simulink model "PlanControlZW_cs"  (R2020a)
settings: Solver=VariableStepAuto  StartTime=0.0  StopTime=100  FixedStep=1/1000  RelTol=1e-3
PreLoadFcn:
  | mbxruntime.callbacks.PreLoadFcn(bdroot);
PostLoadFcn:
  | mbxruntime.callbacks.PostLoadFcn(bdroot);
InitFcn:
  | mbxruntime.callbacks.InitFcn(bdroot);
StartFcn:
  | mbxruntime.callbacks.StartFcn(bdroot);
StopFcn:
  | mbxruntime.callbacks.StopFcn(bdroot);
model workspace (MAT data in the model file):
  mbox_table : object (value not decoded)
  model_closed = 0
  sim_status = 0
values from neighbouring files (symbols this model uses):
  c_factor = 43.75    [emplanner_init.m]
  cf = -175016    [emplanner_init.m]
  cr = -130634    [emplanner_init.m]
  global_path_x = [-2.22044604925e-16 0.999382255067 1.99750536558 2.99435224935 3.98991712279 4.98419835808 5.97719585569 6.96891007764 7.95934169183 8.94849144113 9.93636009523 10.9229484329 ... (501 elements, 501x1)]    [global_Path.mat]
  global_path_y = [-1.75 -1.75 -1.75 -1.75 -1.75 -1.75 -1.75 -1.75 -1.75 -1.75 -1.75 -1.75 ... (501 elements, 501x1)]    [global_Path.mat]
  KD_PID_distance = 0.0    (= 0)    [emplanner_init.m]
  KD_PID_speed = 0    [emplanner_init.m]
  KI_PID_distance = 0.0    (= 0)    [emplanner_init.m]
  KI_PID_speed = 0    [emplanner_init.m]
  KP_PID_distance = 0.5    [emplanner_init.m]
  KP_PID_speed = 1.8    [emplanner_init.m]
  la = 1.265    [emplanner_init.m]
  lb = 2.947-1.265    (= 1.682)    [emplanner_init.m]
  LQR_K1 = k(:,1)'    [emplanner_init.m]
  LQR_K2 = k(:,2)'    [emplanner_init.m]
  LQR_K3 = k(:,3)'    [emplanner_init.m]
  LQR_K4 = k(:,4)'    [emplanner_init.m]
  m = 2020    [emplanner_init.m]
  rack_displacement = [-39.14 , -37.2 , -35.29 , -33.43 , -31.6 , -29.81 , -28.06 , -26.34 , -24.66 ,      -23.01 , -21.38 , -19.79 , -18.23 , -16.69 , -15.18 , -13.7 , -12.23 , -10.8 , -9.38 , -7.98 ,     -6.61 , -5.25 , -3.91 , -2.59 , -1.29 , 0 , 1.27 , 2.54 , 3.78 , 5.02 , 6.24 , 7.46 , 8.66 ,      9.86 , 11.05 , 12.24 , 13.41 , 14.59 , 15.76 , 16.92 , 18.09 , 19.25 , 20.42 , 21.59 , 22.76 ,      23.93 , 25.11 , 26 ...(+26 chars)    [emplanner_init.m]
  refrence_path_x = [2.22044604925e-16 0.999382255067 1.99750536558 2.99435224935 3.98991712279 4.98419835808 5.97719585569 6.96891007764 7.95934169183 8.94849144113 9.93636009523 10.9229484329 ... (501 elements, 501x1)]    [refrence_path_two.mat]
  refrence_path_y = [1.75 1.75 1.75 1.75 1.75 1.75 1.75 1.75 1.75 1.75 1.75 1.75 ... (501 elements, 501x1)]    [refrence_path_two.mat]
  right_wheel_ground = [-70 ,-67.2 , -64.4 , -61.6 , -58.8 , -56 , -53.2 , -50.4 , -47.6 , -44.8 , -42 ,      -39.2 , -36.4 , -33.6 , -30.8 , -28 , -25.2 , -22.4 , -19.6 , -16.8 , -14 , -11.2 , -8.4 , -5.6 ,      -2.8 , 0 , 2.8 , 5.6 , 8.4 , 11.2 , 14 , 16.8 , 19.6 , 22.4 , 25.2 , 28 , 30.8 , 33.6 , 36.4 ,      39.2 , 42 , 44.8 , 47.6 , 50.4 , 53.2 , 56 , 58.8 , 61.6 , 64.4 , 67.2 , 70 ]    [emplanner_init.m]
  vx_break_point = zeros(1,5000)    [emplanner_init.m]
undefined symbols (not defined in the file or in its folder): aubr, DiscIntNeverNeededParam, tablebr, vubr
libraries: PreScanSimulinkLibrary x34, simulink_extras x5, Solver_SF x1
(part 10 of 10)

== matlab function PlanControlZW_cs/Audi_A8_Sedan_1/decision&planning module/EM Planner/speed decision with dynamic planning(dp) ==
  data: obs_st_s_in_set input; dp_speed_s output; obs_st_s_out_set input; obs_st_t_in_set input; obs_st_t_out_set input; dp_speed_t output; reference_speed_unlimit input; w_cost_ref_speed input; w_cost_accel input; w_cost_obs input; plan_start_s_dot input
function [dp_speed_s,dp_speed_t] = fcn(obs_st_s_in_set,obs_st_s_out_set,obs_st_t_in_set,obs_st_t_out_set,reference_speed_unlimit...
    ,w_cost_ref_speed,w_cost_accel,w_cost_obs,plan_start_s_dot)
% 速度动态规划
% 时间从0到8开始规划，最多8秒
% s的范围从0开始到路径规划的path的总长度为止
% 为了减少算力 采用非均匀采样，s越小的越密，越大的越稀疏

s_list = [0:0.5:4.5,...
          5.5:1:14.5,...
          16:1.5:29.5,...
          32:2.5:54.5];
% t 采用均匀采样每 0.5s采样一个点
t_list = 0.5:0.5:8;
% 声明st代价矩阵，表示从起点开始到(i,j)点的最小代价为dp_st_cost(i,j)
% s 采样40个 t 采样 16个 一共是 40 * 16
dp_st_cost = ones(40,16) * inf; % 首先初始化为无穷大
% dp_st_s_dot，表示从起点开始到(i,j)点的最优路径的末速度
dp_st_s_dot = zeros(40,16);
% 需要一个矩阵保持最优路径的前一个节点方便回溯
% dp_st_node(i,j) 表示位置为(i,j)的节点中，最优的上一层节点的行号为dp_st_node(i,j)
dp_st_node = zeros(40,16);
% 计算从dp起点到第一列的cost
for i = 1:length(s_list)
    dp_st_cost(i,1) = CalcDpCost(0,0,i,1,obs_st_s_in_set,obs_st_s_out_set,obs_st_t_in_set,obs_st_t_out_set,...
    w_cost_ref_speed,reference_speed_unlimit,w_cost_accel,w_cost_obs,plan_start_s_dot,s_list,t_list,dp_st_s_dot);
    % 计算第一列所有节点的的s_dot，并存储到dp_st_s_dot中
    % 第一列的前一个节点只有起点，起点的s t 都是0
    [s_end,t_end] = CalcSTCoordinate(i,1,s_list,t_list);
    dp_st_s_dot(i,1) = s_end / t_end;
end
% 动态规划主程序
for i = 2:length(t_list)
    % i 为列循环
    for j = 1:length(s_list)
        % j 为行循环
        % 当前行为 j 列为 i
        cur_row = j;
        cur_col = i;
        % 遍历前一列
        for k = 1:length(s_list)
            pre_row = k;
            pre_col = i - 1;
            % 计算边的代价 其中起点为pre_row,pre_col 终点为cur_row cur_col
            cost_temp = CalcDpCost(pre_row,pre_col,cur_row,cur_col,obs_st_s_in_set,obs_st_s_out_set,...
                obs_st_t_in_set,obs_st_t_out_set,w_cost_ref_speed,reference_speed_unlimit,w_cost_accel,w_cost_obs,...
                plan_start_s_dot,s_list,t_list,dp_st_s_dot);
            if cost_temp + dp_st_cost(pre_row,pre_col) < dp_st_cost(cur_row,cur_col)
                dp_st_cost(cur_row,cur_col) = cost_temp + dp_st_cost(pre_row,pre_col);
                % 计算最优的s_dot
                [s_start,t_start] = CalcSTCoordinate(pre_row,pre_col,s_list,t_list);
                [s_end,t_end] = CalcSTCoordinate(cur_row,cur_col,s_list,t_list);
                dp_st_s_dot(cur_row,cur_col) = (s_end - s_start) / (t_end - t_start);
                % 将最短路径的前一个节点的行号记录下来
                dp_st_node(cur_row,cur_col) = pre_row;
            end      
        end
    end
end
% 输出初始化
dp_speed_s = ones(length(t_list),1) * nan;
dp_speed_t = dp_speed_s;
% 找到dp_node_cost 上边界和右边界代价最小的节点
min_cost = inf;
min_row = inf;
min_col = inf;
% for i = 1:length(s_list)
%     % 遍历右边界
%     if dp_st_cost(i,length(t_list)) <= min_cost
%         min_cost = dp_st_cost(i,length(t_list));
%         min_row = i;
%         min_col = length(t_list);
%     end
% end

for j = 1:length(t_list)-5
    % 遍历上边界
    if dp_st_cost(1,j) <= min_cost
        min_cost = dp_st_cost(1,j);
        min_row = 1;
        min_col = j;
    end
end
% 这里要注意，虽然我们在t上每0.5s采样一个时间，采了16个点，但是min_col 未必等于16
% 也就是说动态规划的最优解的时间未必是8秒
% 所以我们动态规划最后的输出s t 不一定是写满
% 先把终点的ST输出出来
[dp_speed_s(min_col),dp_speed_t(min_col)] = CalcSTCoordinate(min_row,min_col,s_list,t_list);
% 反向回溯
while min_col ~= 1
    pre_row = dp_st_node(min_row,min_col);
    pre_col = min_col - 1;
    [dp_speed_s(pre_col),dp_speed_t(pre_col)] = CalcSTCoordinate(pre_row,pre_col,s_list,t_list);
    min_row = pre_row;
    min_col = pre_col;
end


end

function cost = CalcDpCost(row_start,col_start,row_end,col_end,obs_st_s_in_set,obs_st_s_out_set,obs_st_t_in_set,obs_st_t_out_set,...
    w_cost_ref_speed,reference_speed,w_cost_accel,w_cost_obs,plan_start_s_dot,s_list,t_list,dp_st_s_dot)
    % 该函数将计算链接两个节点之间边的代价
    % 输入：边的起点的行列号row_start,col_start 边的终点行列号row_end,col_end
          % 障碍物st信息obs_st_s_in_set,obs_st_s_out_set,obs_st_t_in_set,obs_st_t_out_set
          % 推荐速度代价权重w_cost_ref_speed,加速度代价权重w_cost_accel,障碍物代价权重w_cost_obs
          % 推荐速度reference_speed
          % 拼接起点的速度plan_start_s_dot
          % s_list,t_list 采样距离
          % dp_st_s_dot 用于计算加速度
    % 首先计算终点的st坐标
    [s_end,t_end] = CalcSTCoordinate(row_end,col_end,s_list,t_list);
    % 规定起点的行列号为0 
    if row_start == 0
        % 边的起点为dp的起点
        s_start = 0;
        t_start = 0;
        s_dot_start = plan_start_s_dot;
    else
        % 边的起点不是dp的起点
        [s_start,t_start] = CalcSTCoordinate(row_start,col_start,s_list,t_list);
        s_dot_start = dp_st_s_dot(row_start,col_start);
    end
    cur_s_dot = (s_end - s_start) / (t_end - t_start);
    cur_s_dot2 = (cur_s_dot - s_dot_start)/(t_end - t_start);
    % 计算推荐速度代价
    cost_ref_speed = w_cost_ref_speed * (cur_s_dot - reference_speed)^2;
    % 计算加速度代价，这里注意，加速度不能超过车辆动力学上下限
    if cur_s_dot2 < 4 && cur_s_dot2 > -6
        cost_accel = w_cost_accel * cur_s_dot2^2;
    else
        % 超过车辆动力学限制，代价会增大很多倍
        cost_accel = 100000 * w_cost_accel * cur_s_dot2^2;
    end
    cost_obs = CalcObsCost(s_start,t_start,s_end,t_end,obs_st_s_in_set,obs_st_s_out_set,obs_st_t_in_set,obs_st_t_out_set,w_cost_obs);
    cost = cost_obs + cost_accel + cost_ref_speed;
end

function obs_cost = CalcObsCost(s_start,t_start,s_end,t_end,obs_st_s_in_set,obs_st_s_out_set,obs_st_t_in_set,obs_st_t_out_set,w_cost_obs)
% 该函数将计算边的障碍物代价
% 输入：边的起点终点s_start,t_start,s_end,t_end
%       障碍物信息 obs_st_s_in_set,obs_st_s_out_set,obs_st_t_in_set,obs_st_t_out_set
%       障碍物代价权重w_cost_obs
% 输出：边的障碍物代价obs_cost
  % 输出初始化
  obs_cost = 0;
  % 采样点的个数
  n = 5;
  % 采样时间间隔
  dt = (t_end - t_start)/(n - 1);
  % 边的斜率
  k = (s_end - s_start)/(t_end - t_start);
  for i = 1:n
      % 计算采样点的坐标
      t = t_start + (i - 1) * dt;
      s = s_start + k * (i - 1) * dt;
      % 遍历所有障碍物
      for j = 1:length(obs_st_s_in_set)
          if isnan(obs_st_s_in_set(j))
              continue;
          end
          % 计算点到st线段的最短距离
          vector1 = [obs_st_s_in_set(j);obs_st_t_in_set(j)] - [s;t];
          vector2 = [obs_st_s_out_set(j);obs_st_t_out_set(j)] - [s;t];
          vector3 = vector2 - vector1;
          min_dis = 0;
          dis1 = sqrt(vector1'*vector1);
          dis2 = sqrt(vector2'*vector2);
          dis3 = abs(vector1(1)*vector3(2) - vector1(2)*vector3(1))/sqrt(vector3'*vector3);
          if (vector1'*vector3 > 0 && vector2'*vector3 > 0) || (vector1'*vector3 < 0 && vector2'*vector3 < 0)
              min_dis = min(dis1,dis2);
          else
              min_dis = dis3;
          end
          obs_cost = obs_cost + CalcCollisionCost(w_cost_obs,min_dis); 
      end
  end
      
end

function collision_cost = CalcCollisionCost(w_cost_obs,min_dis)
  if abs(min_dis) < 0.5
      collision_cost = w_cost_obs;
  elseif abs(min_dis) > 0.5 && abs(min_dis) < 1.5
      % min_dis = 0.5    collision_cost = w_cost_obs^1;
      % min_dis = 1.5    collision_cost = w_cost_obs^0 = 1
      collision_cost = w_cost_obs^((0.5 - min_dis) + 1);
  else
      collision_cost = 0;
  end
end

function [s_value,t_value] = CalcSTCoordinate(row,col,s_list,t_list)
% 该函数将计算矩阵节点的s t 坐标
% 输入 row col 节点在矩阵的行号和列号
%      s_list t_list 采样间隔表
% 输出：s_value t_value 节点的 s t坐标
% 矩阵的(1,1) 代表的是最左上角的元素 s 最大 t 最小
% * 。。。。。。。。
% * 。。。。。。。。
% * 。。。。。。。。
% * 。。。。。。。。
% *****************

% 首先取出矩阵的行数
m = length(s_list);
% 1 1 对应的是 s 的最大值 t 的最小值
s_value = s_list(m - row + 1);
t_value = t_list(col);
end

== matlab function PlanControlZW_cs/Audi_A8_Sedan_1/decision&planning module/EM Planner/generate convex space ==
  data: dp_speed_s input; s_lb output; dp_speed_t input; path_index2s input; obs_st_s_in_set input; obs_st_s_out_set input; obs_st_t_in_set input; obs_st_t_out_set input; s_ub output; s_dot_lb output; s_dot_ub output; trajectory_kappa_init input; max_lateral_accel input
function [s_lb,s_ub,s_dot_lb,s_dot_ub] = fcn(dp_speed_s,dp_speed_t,path_index2s,obs_st_s_in_set,obs_st_s_out_set,...
    obs_st_t_in_set,obs_st_t_out_set,trajectory_kappa_init,max_lateral_accel)
% 该函数将计算出s,s_dot的上下界，开辟凸空间供二次规划使用
% dp_speed_s t 最多有16个，输出初始化n = 16
n = 16;
s_lb = ones(n,1)*-inf;
s_ub = ones(n,1)*inf;
s_dot_lb = ones(n,1)*-inf;
s_dot_ub = ones(n,1)*inf;
path_index2s_end_index = length(path_index2s);
dp_speed_end_index = length(dp_speed_s);

% path_index2s也是有缓冲的，找到有效的path_index2s的末尾的位置，赋值给path_index2s_end_index
for k = 2:length(path_index2s)
    if path_index2s(k) == 0 && path_index2s(k-1) ~= 0
        path_index2s_end_index = k - 1;
        break;
    end
    path_index2s_end_index = k;
end
% 找到dp_speed_s中有效的位置，赋值给dp_speed_end_index
for k = 1:length(dp_speed_s)
    if isnan(dp_speed_s(k))
        dp_speed_end_index = k - 1;
        break;
    end
end

for i = 1:n
    % 该循环将施加车辆动力学约束
    if isnan(dp_speed_s(i))
        break;
    end
    cur_s = dp_speed_s(i);
    % 通过插值的方式找到cur_s 所对应的曲率
    cur_kappa = interp1(path_index2s(1:path_index2s_end_index),trajectory_kappa_init(1:path_index2s_end_index),cur_s);
    % a = v^2 * k => v^2 = a/k 注意除0保护
    max_speed =  sqrt(max_lateral_accel / (abs(cur_kappa) + 1e-10));
    min_speed = 0;
    s_dot_lb(i) = min_speed;
    s_dot_ub(i) = max_speed;    
end



for i = 1:length(obs_st_s_in_set)
    if isnan(obs_st_s_in_set(i))
        continue;
    end
    % 取s t 直线的中点，作为obs_s obs_t 的坐标 
    obs_t = (obs_st_t_in_set(i) + obs_st_t_out_set(i)) / 2;
    obs_s = (obs_st_s_in_set(i) + obs_st_s_out_set(i)) / 2;
    % 计算障碍物的纵向速度
    obs_speed = (obs_st_s_out_set(i) - obs_st_s_in_set(i)) / (obs_st_t_out_set(i) - obs_st_t_in_set(i));
    % 插值找到当t = obs_t时，dp_speed_s 的值
    dp_s = interp1([0;dp_speed_t(1:dp_speed_end_index)],[0;dp_speed_s(1:dp_speed_end_index)],obs_t);
    % 找到dp_speed_t中 与obs_st_t_in_set(i)最近的时间，并将此时间的编号赋值给t_lb_index
    for j = 1:length(dp_speed_t) - 1
        if dp_speed_t(1) > obs_st_t_in_set(i)
            % 如果障碍物切入时间比0.5秒还要短，那么t_lb_index = 1
            break;
        elseif dp_speed_t(j) <= obs_st_t_in_set(i) && dp_speed_t(j + 1) > obs_st_t_in_set(i)
            % 否则遍历dp_speed_t 找到与obs_st_t_in_set(i)最近的点的编号
            break;
        end
    end
    t_lb_index = j;% 将点的编号赋值给j
     % 找到dp_speed_t中 与obs_st_t_out_set(i)最近的时间，并将此时间的编号赋值给t_ub_index
    for j = 1:length(dp_speed_t) - 1
        if dp_speed_t(1) > obs_st_t_out_set(i)
            break;
        elseif dp_speed_t(j) <= obs_st_t_out_set(i) && dp_speed_t(j + 1) > obs_st_t_out_set(i)
            break;
        end
    end
    t_ub_index = j;
    % 这里稍微做个缓冲，把 t_lb_index 稍微缩小一些，t_ub_index稍微放大一些
    t_lb_index = max(t_lb_index - 2,3);% 最低为3 因为碰瓷没法处理
    t_ub_index = min(t_ub_index + 2,dp_speed_end_index);
    if obs_s > dp_s
        % 决策为减速避让
        for m = t_lb_index:t_ub_index
            % 在t_lb_index:t_ub_index的区间上 s的上界不可以超过障碍物st斜直线
            dp_t = dp_speed_t(m);
            s_ub(m) = min(s_ub(m),obs_st_s_in_set(i) + obs_speed * (dp_t - obs_st_t_in_set(i)));
        end
    else 
        % 决策为加速超车
        for m = t_lb_index:t_ub_index
             % 在t_lb_index:t_ub_index的区间上 s的下界不能小于障碍物st斜直线
            dp_t = dp_speed_t(m);
            s_lb(m) = max(s_lb(m),5+obs_st_s_in_set(i) + obs_speed * (dp_t - obs_st_t_in_set(i)));
        end
    end
        
end

== matlab function PlanControlZW_cs/Audi_A8_Sedan_1/decision&planning module/EM Planner/MATLAB Function5 ==
  data: dp_speed_s input; dp_speed_t input; qp_speed_s input; qp_speed_t input; obs_s_in_set input; obs_s_out_set input; obs_t_in_set input; obs_t_out_set input
function  fcn(dp_speed_s,dp_speed_t,qp_speed_s,qp_speed_t,obs_s_in_set,obs_s_out_set,obs_t_in_set,obs_t_out_set)
coder.extrinsic("plot");
cla;
n = length(dp_speed_s);
m = length(obs_s_in_set);
s = length(qp_speed_s);
for i = 1:length(dp_speed_s)
    if isnan(dp_speed_s(i))
        n = i -1;
        break;
    end
end
for i = 1:length(qp_speed_s)
    if isnan(qp_speed_s(i))
        s = i -1;
        break;
    end
end

plot(dp_speed_t(1:n),dp_speed_s(1:n),'r')
plot(qp_speed_t(1:s),qp_speed_s(1:s),'b')
hold on
axis([-1 10 -10 150]);
for i = 1:m
    if isnan(obs_s_in_set(i))
        continue;
    end
    point_t = [obs_t_in_set(i),obs_t_out_set(i)];
    point_s = [obs_s_in_set(i),obs_s_out_set(i)];
    plot(point_t,point_s)
end

== matlab function PlanControlZW_cs/Audi_A8_Sedan_1/decision&planning module/EM Planner/spee planning with quadratic programming (qp) ==
  data: plan_start_s_dot input; qp_s_init output; plan_start_s_dot2 input; dp_speed_s input; dp_speed_t input; s_lb input; s_ub input; s_dot_lb input; s_dot_ub input; qp_s_dot_init output; qp_s_dot2_init output; relative_time_init output; w_cost_s_dot2 input; w_cost_v_ref input; w_cost_jerk input; speed_reference input
function [qp_s_init,qp_s_dot_init,qp_s_dot2_init,relative_time_init] = fcn(plan_start_s_dot,...
    plan_start_s_dot2,dp_speed_s,dp_speed_t,s_lb,s_ub,s_dot_lb,s_dot_ub,w_cost_s_dot2,w_cost_v_ref,w_cost_jerk,speed_reference)
%速度二次规划
% 输入：规划起点plan_start_s_dot,plan_start_s_dot2
%       动态规划结果dp_speed_s,dp_speed_t
%       凸空间约束 s_lb,s_ub,s_dot_lb,s_dot_ub
%       加速度代价权重，推荐速度代价权重，jerk代价权重w_cost_s_dot2,w_cost_v_ref,w_cost_jerk
%       参考速度speed_reference
% 输出：速度曲线qp_s_init,qp_s_dot_init,qp_s_dot2_init,relative_time_init
coder.extrinsic("quadprog")
% 由于dp的结果未必是16，该算法将计算dp_speed_end到底是多少
dp_speed_end = 16;
for i = 1:length(dp_speed_s)
    
    if isnan(dp_speed_s(i))
        dp_speed_end = i - 1;
        break;
    end
end
% 由于dp_speed_end实际上是不确定的，但是输出要求必须是确定长度的值，因此
% 输出初始化选择dp_speed_end的最大值 + 规划起点作为输出初始化的规模
n = 17;

qp_s_init = ones(n,1) * nan;
qp_s_dot_init = ones(n,1) * nan;
qp_s_dot2_init = ones(n,1) * nan;
relative_time_init = ones(n,1) * nan;
s_end = dp_speed_s(dp_speed_end);
% 此时dp_speed_end表示真正有效的dp_speed_t的元素个数，取出dp_speed_t有效的最后一个元素作为规划的时间终点
% 记为recommend_T
recommend_T = dp_speed_t(dp_speed_end);
% qp的规模应该是dp的有效元素的个数 + 规划起点
qp_size = dp_speed_end + 1;
% 连续性约束矩阵初始化，这里的等式约束应该是 Aeq'*X == beq 有转置
Aeq = zeros(3*qp_size,2*qp_size - 2);
beq = zeros(2*qp_size - 2,1);
% 不等式约束初始化
lb = ones(3*qp_size,1);
ub = lb;
% 计算采样间隔时间dt
dt = recommend_T/dp_speed_end;
A_sub =[1,0;
        dt,1;
        (1/3)*dt^2,(1/2)*dt;
        -1,0;
        0,-1;
        (1/6)*dt^2,dt/2];
for i = 1:qp_size - 1
    Aeq(3*i-2:3*i+3,2*i-1:2*i) = A_sub;
end
% 这里初始化不允许倒车约束，也就是 s(i) - s(i+1) <= 0
A = zeros(qp_size-1,3*qp_size);
b = zeros(qp_size-1,1);
for i = 1:qp_size-1
    A(i,3*i - 2) = 1;
    A(i,3*i + 1) = -1;
end
% 由于生成的凸空间约束s_lb s_ub不带起点，所以lb(i) = s_lb(i-1) 以此类推
% 允许最小加速度为-6 最大加速度为4(基于车辆动力学)
for i = 2:qp_size
   lb(3*i - 2) = s_lb(i-1);
   lb(3*i - 1) = s_dot_lb(i-1);
   lb(3*i) = -50;
   ub(3*i - 2) = s_ub(i-1);
   ub(3*i - 1) = s_dot_ub(i-1);
   ub(3*i) = 15;
end
% 起点约束
lb(1) = 0;
lb(2) = plan_start_s_dot;
lb(3) = plan_start_s_dot2;
ub(1) = lb(1);
ub(2) = lb(2);
ub(3) = lb(3);
% 加速度代价 jerk代价 以及推荐速度代价
A_s_dot2 = zeros(3*qp_size,3*qp_size);
A_jerk = zeros(3*qp_size,qp_size - 1);
A_ref = zeros(3*qp_size,3*qp_size);

A4_sub =[0;0;1;0;0;-1];
for i = 1:qp_size
    A_s_dot2(3*i,3*i) = 1;
    A_ref(3*i-1,3*i-1) = 1;
end
for i = 1:qp_size - 1   
   A_jerk(3*i-2:3*i+3,i:i) = A4_sub;
end
% 生成H f
H = w_cost_s_dot2 * (A_s_dot2 * A_s_dot2') + w_cost_jerk * (A_jerk * A_jerk') + w_cost_v_ref * (A_ref * A_ref');
H = 2*H;
f = zeros(3*qp_size,1);
for i = 1:qp_size
    f(3*i-1) =  - 2 * w_cost_v_ref * speed_reference;
end
% 计算二次规划
X = quadprog(H,f,A,b,Aeq',beq,lb,ub);
% 将结果输出
for i = 1:qp_size
   qp_s_init(i) = X(3*i - 2);
   qp_s_dot_init(i) = X(3*i - 1);
   qp_s_dot2_init(i) = X(3*i);
   relative_time_init(i) = (i - 1)*dt;
end

== matlab function PlanControlZW_cs/Audi_A8_Sedan_1/decision&planning module/EM Planner/calc plan start info and stitch trajectory ==
  data: pre_trajectory_x input; plan_start_x output; pre_trajectory_y input; pre_trajectory_heading input; pre_trajectory_kappa input; pre_trajectory_velocity input; pre_trajectory_accel input; pre_trajectory_time input; current_time input; host_x input; host_y input; host_heading_xy input; host_vx input; host_vy input; host_ax input; host_ay input; plan_start_y output; plan_start_heading output; plan_start_kappa output; plan_start_vx output; plan_start_vy output; plan_start_ax output; plan_start_ay output; plan_start_time output; stitch_x output; stitch_y output; stitch_heading output; stitch_kappa output; stitch_speed output; stitch_accel output; stitch_time output
function [plan_start_x,plan_start_y,plan_start_heading,plan_start_kappa,plan_start_vx,plan_start_vy,plan_start_ax,...
    plan_start_ay,plan_start_time,stitch_x,stitch_y,stitch_heading,stitch_kappa,stitch_speed,stitch_accel,stitch_time] ...
    = fcn(pre_trajectory_x,pre_trajectory_y,pre_trajectory_heading,pre_trajectory_kappa,pre_trajectory_velocity,...
    pre_trajectory_accel,pre_trajectory_time,current_time,host_x,host_y,host_heading_xy,host_vx,host_vy,host_ax,host_ay)
%该函数将计算规划的起点以及拼接轨迹的信息
%输入 上一周期的规划结果信息pre_trajectory x ,y,heading,kappa,velocity,accel,time
%     本周期的绝对时间current_time
%     定位信息host x,y,heading,kappa,vx,vy,ax,ay
%输出 规划起点信息plan_start x,y,heading,kappa,vx,vy,ax,ay(vx,vy,ax,ay)是世界坐标系的
%     待拼接的轨迹信息，一般在上一周期的轨迹中的current_time+100ms，往前取20个点。
%     当规划完成后，本周期的规划结果和stitch_trajectory一起拼好发给控制

%输出初始化
stitch_x = zeros(20,1);
stitch_y = zeros(20,1);
stitch_heading = zeros(20,1);
stitch_kappa = zeros(20,1);
stitch_speed = zeros(20,1);
stitch_accel = zeros(20,1);
%时间为负代表没有对应的拼接轨迹
stitch_time = ones(20,1)*-1;

%申明全局变量
persistent is_first_run;
if isempty(is_first_run)
    %代表代码首次运行
    is_first_run = 0;
    %按照轨迹拼接算法，应该用车辆动力学递推，但是首次运行车辆的速度都是0，所以没必要递推了
    plan_start_x = host_x;
    plan_start_y = host_y;
    plan_start_heading = host_heading_xy;
    plan_start_kappa = 0;
    plan_start_vx = 0;
    plan_start_vy = 0;
    plan_start_ax = 0;
    plan_start_ay = 0;
    %规划的起点的时间应该是当前时间+100ms
    plan_start_time = current_time + 0.1;
else
    %该函数不是首次运行
    x_cur = host_x;
    y_cur = host_y;
    heading_cur = host_heading_xy;
    kappa_cur = 0;
    %vx vy ax ay要转换成世界坐标系
    vx_cur = host_vx*cos(heading_cur) - host_vy*sin(heading_cur);
    vy_cur = host_vx*sin(heading_cur) + host_vy*cos(heading_cur);
    ax_cur = host_ax*cos(heading_cur) - host_ay*sin(heading_cur);
    ay_cur = host_ax*sin(heading_cur) + host_ay*cos(heading_cur);
    %规划周期
    dt = 0.1;
    %由于不是首次运行了，有上一时刻的轨迹了，找到上一周期轨迹规划的本周期车辆应该在的位置
    for i = 1:length(pre_trajectory_time) - 1
        if (pre_trajectory_time(i) <= current_time && pre_trajectory_time(i + 1) > current_time)
            break;
        end
    end
    %上一周期规划的本周期的车应该在的位置
    pre_x_desire = pre_trajectory_x(i);
    pre_y_desire = pre_trajectory_y(i);
    pre_heading_desire = pre_trajectory_heading(i);
    %计算横纵向误差
    %切向量
    tor = [cos(pre_heading_desire);sin(pre_heading_desire)];
    %法向量
    nor = [-sin(pre_heading_desire);cos(pre_heading_desire)];
    %误差向量
    d_err = [host_x;host_y] - [pre_x_desire;pre_y_desire];
    %纵向误差
    lon_err = abs(d_err'*tor);
    %横向误差
    lat_err = abs(d_err'*nor);
    %纵向误差大于2.5 横向误差大于0.5 认为控制没跟上
    if (lon_err > 2.5)||(lat_err > 0.5)
        %此分支处理控制未跟上的情况，规划起点通过运动学递推
        plan_start_x = x_cur + vx_cur * dt + 0.5 * ax_cur * dt * dt;
        plan_start_y = y_cur + vy_cur * dt + 0.5 * ay_cur * dt * dt;
        plan_start_vx = vx_cur + ax_cur * dt;
        plan_start_vy = vy_cur + ay_cur * dt;
        plan_start_heading = atan2(plan_start_vy,plan_start_vx);
        plan_start_ax = ax_cur;
        plan_start_ay = ay_cur;
        plan_start_kappa = kappa_cur;
        plan_start_time = current_time + 0.1;
        return;
    else
        %此分支表示控制能跟的上规划，开始拼接
        for j = i:length(pre_trajectory_time) - 1
            if (pre_trajectory_time(j) <= current_time + 0.1)&&(pre_trajectory_time(j + 1) > current_time + 0.1)
                break;
            end
        end
        %注：此算法要能运行需要trajectory的点有很高的密度
        plan_start_x = pre_trajectory_x(j);
        plan_start_y = pre_trajectory_y(j);
        plan_start_heading = pre_trajectory_heading(j);
        plan_start_kappa = pre_trajectory_kappa(j);
        %这里的pre_trajectory的速度,加速度是指轨迹的切向速度，切向加速度
        plan_start_vx = pre_trajectory_velocity(j) * cos(plan_start_heading);
        plan_start_vy = pre_trajectory_velocity(j) * sin(plan_start_heading);
        %控制所跟踪的速度和加速度就是规划的轨迹的速度和切向加速度
        %pre_trajectory的加速度是切向加速度，要想计算ax,ay还要计算法向加速度
        %计算轨迹在current_time + 100ms 这个点的切向量法向量
        tor = [cos(plan_start_heading);sin(plan_start_heading)];
        nor = [-sin(plan_start_heading);cos(plan_start_heading)];
        a_tor = pre_trajectory_accel(j) * tor;
        a_nor = pre_trajectory_velocity(j)^2 * plan_start_kappa * nor ;
        plan_start_ax = a_tor(1) + a_nor(1);
        plan_start_ay = a_tor(2) + a_nor(2);
        plan_start_time = pre_trajectory_time(j);
        %计算拼接轨迹
        %j 表示 current_time + 0.1 的时间点在 pre_trajectory_time的编号
        %拼接是往从j开始，往前拼接20个，也就是pre_trajectory(j-1),j-2,j-3,....j-19
        %分两种情况，如果j小于20，意味着前面的轨迹点不够20个
        %如果j >= 20,意味着前面的点多于20个
        %还有一个细节需要考虑，pre_trajectory x(j) y(j) ....是规划的起点，那么在轨迹拼接时
        %需不需要在stitch_trajectory中把pre_trajectory x(j) y(j) ....包含进去
        %答案是否定的，不应该包进去，因为规划的起点会在规划模块计算完成后的结果中包含，如果在拼接的时候
        %还要包含，那就等于规划起点包含了两次
        %除非本周期计算的轨迹不包含规划起点，那么stitch_trajectory可以包含规划起点。
        %如果本周期计算的轨迹包含规划起点，那么stitch_trajectory就不可以包含规划起点。
        %我们选择规划包含起点，拼接不包含起点的做法
        
        %把起点去掉
        j = j - 1;
        if j >= 20
            stitch_x = pre_trajectory_x(j - 19:j);
            stitch_y = pre_trajectory_y(j - 19:j);
            stitch_heading = pre_trajectory_heading(j - 19:j);
            stitch_kappa = pre_trajectory_kappa(j - 19:j);
            stitch_speed = pre_trajectory_velocity(j - 19:j);
            stitch_accel = pre_trajectory_accel(j - 19:j);
            stitch_time = pre_trajectory_time(j - 19:j);
        else
            stitch_x(20 - j + 1:20) = pre_trajectory_x(1:j);
            stitch_y(20 - j + 1:20) = pre_trajectory_y(1:j);
            stitch_heading(20 - j + 1:20) = pre_trajectory_heading(1:j);
            stitch_kappa(20 - j + 1:20) = pre_trajectory_kappa(1:j);
            stitch_speed(20 - j + 1:20) = pre_trajectory_velocity(1:j);
            stitch_accel(20 - j + 1:20) = pre_trajectory_accel(1:j);
            stitch_time(20 - j + 1:20) = pre_trajectory_time(1:j);           
        end   
    end    
end

== matlab function PlanControlZW_cs/Audi_A8_Sedan_1/decision&planning module/EM Planner/path planning task1/path planning with quadratic programming (qp) ==
  data: qp_path_s output; l_min input; qp_path_l output; l_max input; w_cost_l input; w_cost_dl input; w_cost_ddl input; w_cost_dddl input; w_cost_centre input; w_cost_end_l input; w_cost_end_dl input; w_cost_end_ddl input; host_d1 input; host_d2 input; host_w input; plan_start_s input; plan_start_l input; plan_start_dl input; plan_start_ddl input; qp_path_dl output; qp_path_ddl output; delta_dl_max input; delta_ddl_max input; dp_path_l_final input
function [qp_path_s,qp_path_l,qp_path_dl,qp_path_ddl] = ...
fcn(l_min,l_max,w_cost_l,w_cost_dl,w_cost_ddl,w_cost_dddl,w_cost_centre,w_cost_end_l,w_cost_end_dl,w_cost_end_ddl,...
    host_d1,host_d2,host_w,...
    plan_start_s,plan_start_l,plan_start_dl,plan_start_ddl,...
    delta_dl_max,delta_ddl_max,dp_path_l_final)
% 路径二次规划
% 0.5*x'Hx + f'*x = min
% subject to A*x <= b
%            Aeq*x = beq
%            lb <= x <= ub;
% 输入：l_min l_max 点的凸空间
%       w_cost_l 参考线代价
%       w_cost_dl ddl dddl 光滑性代价
%       w_cost_centre 凸空间中央代价
%       w_cost_end_l dl dd1 终点的状态代价 (希望path的终点状态为(0,0,0))
%       host_d1,d2 host质心到前后轴的距离
%       host_w host的宽度
%       plan_start_l,dl,ddl 规划起点
% 输出 qp_path_l dl ddl 二次规划输出的曲线
coder.extrinsic("quadprog");
% 待优化的变量的数量
n = 20;

% 输出初始化
qp_path_l = zeros(n,1);
qp_path_dl = zeros(n,1);
qp_path_ddl = zeros(n,1);
qp_path_s = zeros(n,1);

% H_L H_DL H_DDL H_DDDL Aeq beq A b 初始化
H_L = zeros(3*n, 3*n);
H_DL = zeros(3*n, 3*n);
H_DDL = zeros(3*n, 3*n);
H_DDDL = zeros(n-1, 3*n);
H_CENTRE = zeros(3*n, 3*n);
H_L_END = zeros(3*n, 3*n);
H_DL_END = zeros(3*n, 3*n);
H_DDL_END = zeros(3*n, 3*n);
Aeq = zeros(2*n-2, 3*n);
beq = zeros(2*n-2, 1);
A = zeros(8*n, 3*n);
b = zeros(8*n, 1);
% 更新：加入 dl(i+1) - dl(i) ddl(i+1) - ddl(i) 的约束
A_dl_minus = zeros(n - 1,3*n);
b_dl_minus = zeros(n - 1,1);
A_ddl_minus = zeros(n - 1,3*n);
b_ddl_minus = zeros(n - 1,1);
for i = 1:n-1
    row = i;
    col = 3*i - 2;
    A_dl_minus(row,col:col+5) = [0 -1 0 0 1 0];
    b_dl_minus(row) = delta_dl_max;
    A_ddl_minus(row,col:col+5) = [0 0 -1 0 0 1];
    b_ddl_minus(row) = delta_ddl_max;
end
% -max < a*x < max => ax < max && -ax < -(-max)
A_minus = [A_dl_minus;
          -A_dl_minus;
           A_ddl_minus;
          -A_ddl_minus];
b_minus = [b_dl_minus;
           b_dl_minus;
          b_ddl_minus;
          b_ddl_minus]; 

%  期望的终点状态
end_l_desire = 0;
end_dl_desire = 0;
end_ddl_desire = 0;

% Aeq_sub
ds = 3;%纵向间隔
for i = 1:n
    qp_path_s(i) = plan_start_s + (i-1)*ds;
end

Aeq_sub = [1 ds ds^2/3 -1 0 ds^2/6;
           0 1  ds/2   0 -1 ds/2];
% A_sub;
d1 = host_d1;
d2 = host_d2;
w = host_w;
A_sub = [1  d1 0;
         1  d1 0;
         1 -d2 0;
         1 -d2 0;
        -1 -d1 0;
        -1 -d1 0;
        -1  d2 0;
        -1  d2 0];
% 生成Aeq
for i = 1:n-1
    % 计算分块矩阵左上角的行和列
    row = 2*i - 1;
    col = 3*i - 2;
    Aeq(row:row + 1,col:col + 5) = Aeq_sub;
end
% 生成A
for i = 2:n
    row = 8*i - 7;
    col = 3*i - 2;
    A(row:row + 7,col:col + 2) = A_sub;
end

% 视频里用的找(s(i) - d2,s(i) + d1)的方法过于保守，在这里舍弃掉
% 只要找到四个角点所对应的l_min l_max 即可
% 。。。。。。。。。。。。。。
%    [    .   ]<- 
%    [        ]
% 。。。。。。。。。。。。。
front_index = ceil(d1/ds);
back_index = ceil(d2/ds); % ceil向上取整 ceil(3) = 3 ceil(3.1) = 4
% 生成b
for i = 2:n
    % 左前 右前的index = min(i + front_index,60)
    % 左后 右后的index = max(i - back_index,1)
    % l_min l_max 都是60个点
    index1 = min(3*i - 2 + front_index,n);
    index2 = max(3*i - 2 - back_index,1);
    b(8*i - 7:8*i,1) = [l_max(index1) - w/2;
                        l_max(index1) + w/2;
                        l_max(index2) - w/2;
                        l_max(index2) + w/2;
                       -l_min(index1) + w/2;
                       -l_min(index1) - w/2;
                       -l_min(index2) + w/2;
                       -l_min(index2) - w/2;];
end
%生成 lb ub 主要是对规划起点做约束
lb = ones(3*n,1)*-inf;
ub = ones(3*n,1)*inf;
lb(1) = plan_start_l;
lb(2) = plan_start_dl;
lb(3) = plan_start_ddl;
ub(1) = lb(1);
ub(2) = lb(2);
ub(3) = lb(3);
for i = 2:n
    lb(3*i - 1) = - 2; %约束 l'
    ub(3*i - 1) = 2;
    lb(3*i) = -0.1; %约束 l''
    ub(3*i) = 0.1;
end
% 生成H_L,H_DL,H_DDL,H_CENTRE
for i = 1:n
    H_L(3*i - 2,3*i - 2) = 1;
    H_DL(3*i - 1,3*i - 1) = 1;
    H_DDL(3*i, 3*i) = 1;
end
H_CENTRE = H_L;
% 生成H_DDDL;
H_dddl_sub = [0 0 1 0 0 -1];
for i = 1:n-1
    row = i;
    col = 3*i - 2;
    H_DDDL(row,col:col + 5) = H_dddl_sub;
end
% 生成H_L_END H_DL_END H_DDL_END
H_L_END(3*n - 2,3*n - 2) = 1;
H_DL_END(3*n - 1,3*n - 1) = 1;
H_DDL_END(3*n,3*n) = 1;
% 生成二次规划的H 因为ds ！= 1 所以 dddl = delta_ddl/ds;
H = w_cost_l * (H_L'*H_L) + w_cost_dl * (H_DL'*H_DL) + w_cost_ddl * (H_DDL'*H_DDL)...
   +w_cost_dddl * (H_DDDL'*H_DDDL)/ds + w_cost_centre * (H_CENTRE'*H_CENTRE) + w_cost_end_l * (H_L_END'*H_L_END)...
   +w_cost_end_dl * (H_DL_END'* H_DL_END) + w_cost_ddl * (H_DDL_END'*H_DDL_END);
H = 2 * H;
% 生成f
f = zeros(3*n,1);
% centre_line = 0.5 * (l_min + l_max); % 此时centre line 还是60个点
centre_line = dp_path_l_final+0.3;
for i = 1:n
    f(3*i - 2) = -2 * centre_line(3*i - 2);
end
% 避免centreline权重过大影响轨迹平顺性
for i = 1:n
    if abs(f(i)) > 0.3
        f(i) = w_cost_centre * f(i);
    end
end
% 终点要接近end_l dl ddl desire
f(3*n - 2) = f(3*n - 2) -2 * end_l_desire * w_cost_end_l;
f(3*n - 1) = f(3*n - 1) -2 * end_dl_desire * w_cost_end_dl;
f(3*n) = f(3*n) -2 * end_ddl_desire * w_cost_end_ddl;

X = quadprog(H,f,A,b,Aeq,beq,lb,ub);

for i = 1:n
    qp_path_l(i) = X(3*i - 2);
    qp_path_dl(i) = X(3*i - 1);
    qp_path_ddl(i) = X(3*i);
end

end

== matlab function PlanControlZW_cs/Audi_A8_Sedan_1/biandao_yitu/MATLAB Function ==
  data: safe_d input; real_x output; global_path_x input; global_path_y input; refrence_path_x input; refrence_path_y input; real_y output
function [real_x,real_y]= fcn(safe_d,global_path_x,global_path_y,refrence_path_x,refrence_path_y)

if safe_d>30
  real_x=global_path_x;
  real_y=global_path_y;
else
     real_x=refrence_path_x;
     real_y=refrence_path_y;
end
